simulink model "GraphicEqualizer"  (Simulink 6.6)
settings: Solver=FixedStepDiscrete  StartTime=0.0  StopTime=inf  RelTol=1e-3
PreLoadFcn:
  | Frame=64;  % number of points in a frame
InitFcn:
  | GraphicGUI
StopFcn:
  | save_system(gcs)
  | save eq_coefficients  num_den_coef
  | GraphicGUI('save_state')
undefined symbols (not defined in the file or in its folder): dfilt
libraries: dspsrcs4 x16, dsparch4 x5, simulink x2, dspwin32 x2
CloseFcn:
  | close all
settings Model: Creator=aanantha  LastModifiedBy=allways
settings DataIOCC: SaveOutput=off  SaveTime=off  SignalLoggingName=sigsOut
settings DebuggingCC: SignalResolutionControl=TryResolveAllWithWarning  SolverPrmCheckMsg=none  InheritedTsInSrcMsg=none  MultiTaskDSMMsg=warning  MultiTaskCondExecSysMsg=none  MultiTaskRateTransMsg=warning  StrictBusMsg=None
settings HardwareCC: TargetUnknown=on
settings RTWCC: IncludeERTFirstTime=on

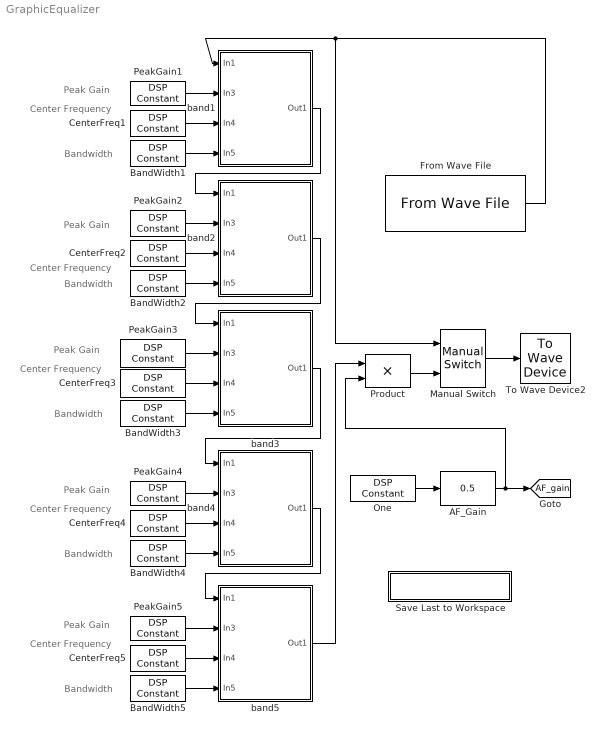
== system GraphicEqualizer ==
  note: Peak Gain
  note: Center Frequency
  note: Bandwidth
  note: Peak Gain
  note: Center Frequency
  note: Bandwidth
  note: Peak Gain
  note: Center Frequency
  note: Bandwidth
  note: Peak Gain
  note: Center Frequency
  note: Bandwidth
  note: Peak Gain
  note: Center Frequency
  note: Bandwidth
  AF_Gain : simulink/Math Operations/Slider Gain  SystemSampleTime=-1  low=0.1  gain=0.5  high=1
  BandWidth1 : dspsrcs4/DSP Constant  Tag=paramsBlock  SystemSampleTime=-1  Value=0.0071238  SampleMode=Discrete  discreteOutput=Sample-based  continuousOutput=Sample-based  sampTime=-1  framePeriod=-1  dataType=Inherit from 'Constant value'  isSigned=on  wordLen=16  udDataType=sfix(16)  fracBitsMode=Best precision  numFracBits=15  InterpretAs1D=off  Ts=-1  FramebasedOutput=off
      settings: AttributesFormatString=\n\n\n\n
  BandWidth2 : dspsrcs4/DSP Constant  Tag=paramsBlock  SystemSampleTime=-1  Value=0.070364  SampleMode=Discrete  discreteOutput=Sample-based  continuousOutput=Sample-based  sampTime=-1  framePeriod=-1  dataType=Inherit from 'Constant value'  isSigned=on  wordLen=16  udDataType=sfix(16)  fracBitsMode=Best precision  numFracBits=15  InterpretAs1D=off  Ts=-1  FramebasedOutput=off
      settings: AttributesFormatString=\n\n\n\n
  BandWidth3 : dspsrcs4/DSP Constant  Tag=paramsBlock  SystemSampleTime=-1  Value=0.66183  SampleMode=Discrete  discreteOutput=Sample-based  continuousOutput=Sample-based  sampTime=-1  framePeriod=-1  dataType=Inherit from 'Constant value'  isSigned=on  wordLen=16  udDataType=sfix(16)  fracBitsMode=Best precision  numFracBits=15  InterpretAs1D=off  Ts=-1  FramebasedOutput=off
      settings: AttributesFormatString=\n\n\n\n
  BandWidth4 : dspsrcs4/DSP Constant  Tag=paramsBlock  SystemSampleTime=-1  Value=0.44704  SampleMode=Discrete  discreteOutput=Sample-based  continuousOutput=Sample-based  sampTime=-1  framePeriod=-1  dataType=Inherit from 'Constant value'  isSigned=on  wordLen=16  udDataType=sfix(16)  fracBitsMode=Best precision  numFracBits=15  InterpretAs1D=off  Ts=-1  FramebasedOutput=off
      settings: AttributesFormatString=\n\n\n\n
  BandWidth5 : dspsrcs4/DSP Constant  Tag=paramsBlock  SystemSampleTime=-1  Value=0.039703  SampleMode=Discrete  discreteOutput=Sample-based  continuousOutput=Sample-based  sampTime=-1  framePeriod=-1  dataType=Inherit from 'Constant value'  isSigned=on  wordLen=16  udDataType=sfix(16)  fracBitsMode=Best precision  numFracBits=15  InterpretAs1D=off  Ts=-1  FramebasedOutput=off
      settings: AttributesFormatString=\n\n\n\n
  CenterFreq1 : dspsrcs4/DSP Constant  Tag=paramsBlock  SystemSampleTime=-1  Value=0.034624  SampleMode=Discrete  discreteOutput=Sample-based  continuousOutput=Sample-based  sampTime=-1  framePeriod=-1  dataType=Inherit from 'Constant value'  isSigned=on  wordLen=16  udDataType=sfix(16)  fracBitsMode=Best precision  numFracBits=15  InterpretAs1D=off  Ts=-1  FramebasedOutput=off
      settings: AttributesFormatString=\n\n\n\n
  CenterFreq2 : dspsrcs4/DSP Constant  Tag=paramsBlock  SystemSampleTime=-1  Value=0.016233  SampleMode=Discrete  discreteOutput=Sample-based  continuousOutput=Sample-based  sampTime=-1  framePeriod=-1  dataType=Inherit from 'Constant value'  isSigned=on  wordLen=16  udDataType=sfix(16)  fracBitsMode=Best precision  numFracBits=15  InterpretAs1D=off  Ts=-1  FramebasedOutput=off
      settings: AttributesFormatString=\n\n\n\n
  CenterFreq3 : dspsrcs4/DSP Constant  Tag=paramsBlock  SystemSampleTime=-1  Value=1.2233  SampleMode=Discrete  discreteOutput=Sample-based  continuousOutput=Sample-based  sampTime=-1  framePeriod=-1  dataType=Inherit from 'Constant value'  isSigned=on  wordLen=16  udDataType=sfix(16)  fracBitsMode=Best precision  numFracBits=15  InterpretAs1D=off  Ts=-1  FramebasedOutput=off
      settings: AttributesFormatString=\n\n\n\n
  CenterFreq4 : dspsrcs4/DSP Constant  Tag=paramsBlock  SystemSampleTime=-1  Value=0.88231  SampleMode=Discrete  discreteOutput=Sample-based  continuousOutput=Sample-based  sampTime=-1  framePeriod=-1  dataType=Inherit from 'Constant value'  isSigned=on  wordLen=16  udDataType=sfix(16)  fracBitsMode=Best precision  numFracBits=15  InterpretAs1D=off  Ts=-1  FramebasedOutput=off
      settings: AttributesFormatString=\n\n\n\n
  CenterFreq5 : dspsrcs4/DSP Constant  Tag=paramsBlock  SystemSampleTime=-1  Value=0.084415  SampleMode=Discrete  discreteOutput=Sample-based  continuousOutput=Sample-based  sampTime=-1  framePeriod=-1  dataType=Inherit from 'Constant value'  isSigned=on  wordLen=16  udDataType=sfix(16)  fracBitsMode=Best precision  numFracBits=15  InterpretAs1D=off  Ts=-1  FramebasedOutput=off
      settings: AttributesFormatString=\n\n\n\n
  From Wave File : dspwin32/From Wave File  FileName=HatikvahClip.wav  SamplesPerFrame=Frame  MinBufSize=256  dType=double  bLoop=on  timesToPlay=inf  restartMode=at beginning of next frame (zero pad)  firstSampleOutput=off  lastSampleOutput=off
  Manual Switch : simulink/Signal Routing/Manual Switch  SystemSampleTime=-1  sw=0  action=0  varsize=off
  One : dspsrcs4/DSP Constant  Tag=paramsBlock  SystemSampleTime=-1  Value=1  SampleMode=Discrete  discreteOutput=Sample-based  continuousOutput=Sample-based  sampTime=-1  framePeriod=-1  dataType=Inherit from 'Constant value'  isSigned=on  wordLen=16  udDataType=sfix(16)  fracBitsMode=Best precision  numFracBits=15  InterpretAs1D=off  Ts=-1  FramebasedOutput=off
      settings: AttributesFormatString=\n\n\n\n
  PeakGain1 : dspsrcs4/DSP Constant  Tag=paramsBlock  SystemSampleTime=-1  Value=-2.5998  SampleMode=Discrete  discreteOutput=Sample-based  continuousOutput=Sample-based  sampTime=-1  framePeriod=-1  dataType=Inherit from 'Constant value'  isSigned=on  wordLen=16  udDataType=sfix(16)  fracBitsMode=Best precision  numFracBits=15  InterpretAs1D=off  Ts=-1  FramebasedOutput=off
      settings: AttributesFormatString=\n\n\n\n
  PeakGain2 : dspsrcs4/DSP Constant  Tag=paramsBlock  SystemSampleTime=-1  Value=-9.6376  SampleMode=Discrete  discreteOutput=Sample-based  continuousOutput=Sample-based  sampTime=-1  framePeriod=-1  dataType=Inherit from 'Constant value'  isSigned=on  wordLen=16  udDataType=sfix(16)  fracBitsMode=Best precision  numFracBits=15  InterpretAs1D=off  Ts=-1  FramebasedOutput=off
      settings: AttributesFormatString=\n\n\n\n
  PeakGain3 : dspsrcs4/DSP Constant  Tag=paramsBlock  SystemSampleTime=-1  Value=-11.0414  SampleMode=Discrete  discreteOutput=Sample-based  continuousOutput=Sample-based  sampTime=-1  framePeriod=-1  dataType=Inherit from 'Constant value'  isSigned=on  wordLen=16  udDataType=sfix(16)  fracBitsMode=Best precision  numFracBits=15  InterpretAs1D=off  Ts=-1  FramebasedOutput=off
      settings: AttributesFormatString=\n\n\n\n
  PeakGain4 : dspsrcs4/DSP Constant  Tag=paramsBlock  SystemSampleTime=-1  Value=8.1249  SampleMode=Discrete  discreteOutput=Sample-based  continuousOutput=Sample-based  sampTime=-1  framePeriod=-1  dataType=Inherit from 'Constant value'  isSigned=on  wordLen=16  udDataType=sfix(16)  fracBitsMode=Best precision  numFracBits=15  InterpretAs1D=off  Ts=-1  FramebasedOutput=off
      settings: AttributesFormatString=\n\n\n\n
  PeakGain5 : dspsrcs4/DSP Constant  Tag=paramsBlock  SystemSampleTime=-1  Value=6.5813  SampleMode=Discrete  discreteOutput=Sample-based  continuousOutput=Sample-based  sampTime=-1  framePeriod=-1  dataType=Inherit from 'Constant value'  isSigned=on  wordLen=16  udDataType=sfix(16)  fracBitsMode=Best precision  numFracBits=15  InterpretAs1D=off  Ts=-1  FramebasedOutput=off
      settings: AttributesFormatString=\n\n\n\n
  Product : Product  SaturateOnIntegerOverflow=on
  Save Last to Workspace : Subsystem
      mask Display: disp('Save Coefficients')
  To Wave Device2 : dspwin32/To Wave Device  bufDuration=2  determineBufSize=on  userIntBufSize=256  initDelay=0.1  useDefaultDevice=off  userDeviceID=SoundMAX HD Audio  enable24Bit=off
  band1 : Subsystem  mask(Parametric Equalizer){G0=0, gbPopup=User-Defined, NdB=.707}
      mask prompts: G0 "Reference gain G0"; gbPopup "Bandwidth Gain"; NdB "Attenuation Factor (Bandwidth Gain = af*Peak Gain; 0<af<1)"
      mask help: This block contains the second order IIR filter which functions as a parametric equalizer. The Inputs to this block, in order, are the Audio In, the peak gain of the equalizer at the center frequency, the center frequency itself, and the bandwidth of the filter around the center frequency. Currently the bandedges are defined as those frequency where the gain falls off to one-half the center frequency peak gain.
      mask StyleString: edit,popup(3 dB(1/2 Power)|User-Defined),edit
      mask CallbackString: |parEqMasking|
      mask Display:
      | port_label ('input',1,'Audio In');
      | port_label ('input',2,'Peak Gain');
      | port_label ('input',3,'Center Frequency');
      | port_label ('input',4,'Bandwidth');
  band2 : Subsystem  mask(Parametric Equalizer){G0=0, gbPopup=User-Defined, NdB=.707}
      mask prompts: G0 "Reference gain G0"; gbPopup "Bandwidth Gain"; NdB "Attenuation Factor (Bandwidth Gain = af*Peak Gain; 0<af<1)"
      mask help: This block contains the second order IIR filter which functions as a parametric equalizer. The Inputs to this block, in order, are the Audio In, the peak gain of the equalizer at the center frequency, the center frequency itself, and the bandwidth of the filter around the center frequency. Currently the bandedges are defined as those frequency where the gain falls off to one-half the center frequency peak gain.
      mask StyleString: edit,popup(3 dB(1/2 Power)|User-Defined),edit
      mask CallbackString: |parEqMasking|
      mask Display:
      | port_label ('input',1,'Audio In');
      | port_label ('input',2,'Peak Gain');
      | port_label ('input',3,'Center Frequency');
      | port_label ('input',4,'Bandwidth');
  band3 : Subsystem  mask(Parametric Equalizer){G0=0, gbPopup=User-Defined, NdB=.707}
      mask prompts: G0 "Reference gain G0"; gbPopup "Bandwidth Gain"; NdB "Attenuation Factor (Bandwidth Gain = af*Peak Gain; 0<af<1)"
      mask help: This block contains the second order IIR filter which functions as a parametric equalizer. The Inputs to this block, in order, are the Audio In, the peak gain of the equalizer at the center frequency, the center frequency itself, and the bandwidth of the filter around the center frequency. Currently the bandedges are defined as those frequency where the gain falls off to one-half the center frequency peak gain.
      mask StyleString: edit,popup(3 dB(1/2 Power)|User-Defined),edit
      mask CallbackString: |parEqMasking|
      mask Display:
      | port_label ('input',1,'Audio In');
      | port_label ('input',2,'Peak Gain');
      | port_label ('input',3,'Center Frequency');
      | port_label ('input',4,'Bandwidth');
  band4 : Subsystem  mask(Parametric Equalizer){G0=0, gbPopup=User-Defined, NdB=.707}
      mask prompts: G0 "Reference gain G0"; gbPopup "Bandwidth Gain"; NdB "Attenuation Factor (Bandwidth Gain = af*Peak Gain; 0<af<1)"
      mask help: This block contains the second order IIR filter which functions as a parametric equalizer. The Inputs to this block, in order, are the Audio In, the peak gain of the equalizer at the center frequency, the center frequency itself, and the bandwidth of the filter around the center frequency. Currently the bandedges are defined as those frequency where the gain falls off to one-half the center frequency peak gain.
      mask StyleString: edit,popup(3 dB(1/2 Power)|User-Defined),edit
      mask CallbackString: |parEqMasking|
      mask Display:
      | port_label ('input',1,'Audio In');
      | port_label ('input',2,'Peak Gain');
      | port_label ('input',3,'Center Frequency');
      | port_label ('input',4,'Bandwidth');
  band5 : Subsystem  mask(Parametric Equalizer){G0=0, gbPopup=User-Defined, NdB=.707}
      mask prompts: G0 "Reference gain G0"; gbPopup "Bandwidth Gain"; NdB "Attenuation Factor (Bandwidth Gain = af*Peak Gain; 0<af<1)"
      mask help: This block contains the second order IIR filter which functions as a parametric equalizer. The Inputs to this block, in order, are the Audio In, the peak gain of the equalizer at the center frequency, the center frequency itself, and the bandwidth of the filter around the center frequency. Currently the bandedges are defined as those frequency where the gain falls off to one-half the center frequency peak gain.
      mask StyleString: edit,popup(3 dB(1/2 Power)|User-Defined),edit
      mask CallbackString: |parEqMasking|
      mask Display:
      | port_label ('input',1,'Audio In');
      | port_label ('input',2,'Peak Gain');
      | port_label ('input',3,'Center Frequency');
      | port_label ('input',4,'Bandwidth');
  tag scope: AF_gain=global
  wires:
  PeakGain2/1 -> band2/2(In3)
  CenterFreq2/1 -> band2/3(In4)
  BandWidth2/1 -> band2/4(In5)
  PeakGain3/1 -> band3/2(In3)
  CenterFreq3/1 -> band3/3(In4)
  BandWidth3/1 -> band3/4(In5)
  From Wave File/1 -> band1/1(In1), Manual Switch/1
  PeakGain1/1 -> band1/2(In3)
  CenterFreq1/1 -> band1/3(In4)
  BandWidth1/1 -> band1/4(In5)
  band1/1(Out1) -> band2/1(In1)
  band2/1(Out1) -> band3/1(In1)
  Manual Switch/1 -> To Wave Device2/1
  One/1 -> AF_Gain/1
  AF_Gain/1 -> Product/2, [AF_gain]
  Product/1 -> Manual Switch/2
  PeakGain4/1 -> band4/2(In3)
  CenterFreq4/1 -> band4/3(In4)
  BandWidth4/1 -> band4/4(In5)
  band4/1(Out1) -> band5/1(In1)
  PeakGain5/1 -> band5/2(In3)
  CenterFreq5/1 -> band5/3(In4)
  BandWidth5/1 -> band5/4(In5)
  band5/1(Out1) -> Product/1
  band3/1(Out1) -> band4/1(In1)

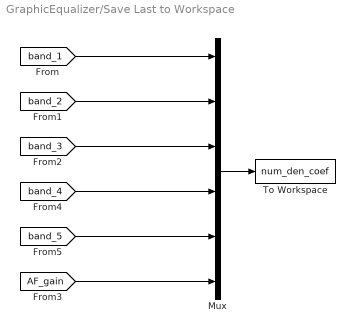
== system GraphicEqualizer/Save Last to Workspace ==
  Mux : Mux  Inputs=6
  To Workspace : ToWorkspace  VariableName=num_den_coef  SampleTime=-1  SaveFormat=Array
      settings: MaxDataPoints=1
  wires:
  [band_2] -> Mux/2
  [band_1] -> Mux/1
  [band_3] -> Mux/3
  Mux/1 -> To Workspace/1
  [band_4] -> Mux/4
  [AF_gain] -> Mux/6
  [band_5] -> Mux/5

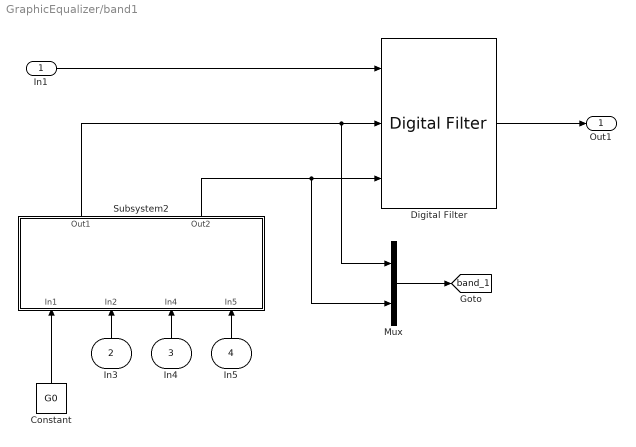
== system GraphicEqualizer/band1 ==
  In1 : Inport
  In3 : Inport  Orientation=up  Port=2
  In4 : Inport  Orientation=up  Port=3
  In5 : Inport  Orientation=up  Port=4
  Constant : Constant  Orientation=up  Value=G0
  Digital Filter : dsparch4/Digital Filter  DialogController=dspdialog.DigitalFilter  DialogControllerArgs=DataTag0  TypePopup=IIR (poles & zeros)  IIRFiltStruct=Direct form II transposed  AllPoleFiltStruct=Direct form  FIRFiltStruct=Direct form  CoeffSource=Input port(s)  NumCoeffs=[1 2]  DenCoeffs=[1 0.1]  BiQuadCoeffs=[1 0.3 0.4 1 0.1 0.2]  LatticeCoeffs=[0.2 0.4]  denIgnore=on  FiltPerSampPopup=One filter per frame  IC=0  ICnum=0  ICden=0  roundingMode=Floor  overflowMode=off  ScaleValues=1  scaleValueFracLength=14  stageInFracLength=15  stageOutFracLength=15  FilterSource=Input port(s)  dfiltObjectName=dfilt.dffir([1 2 1])
  Mux : Mux  Inputs=2
  Subsystem2 : Subsystem  Orientation=up
      mask Display:
      | disp('ParEq')
      | port_label('input',1,'G0');
      | port_label('input',2,'G');
      | port_label('input',3,'w0');
      | port_label('input',4,'Dw');
      | 
      | port_label('output',1,'Num');
      | port_label('output',2,'Den');
  Out1 : Outport
  tag scope: band_1=global
  wires:
  Subsystem2/1(Out1) -> Digital Filter/2, Mux/1
  Subsystem2/2(Out2) -> Digital Filter/3, Mux/2
  In1/1 -> Digital Filter/1
  Digital Filter/1 -> Out1/1
  In3/1 -> Subsystem2/2(In2)
  In4/1 -> Subsystem2/3(In4)
  In5/1 -> Subsystem2/4(In5)
  Constant/1 -> Subsystem2/1(In1)
  Mux/1 -> [band_1]

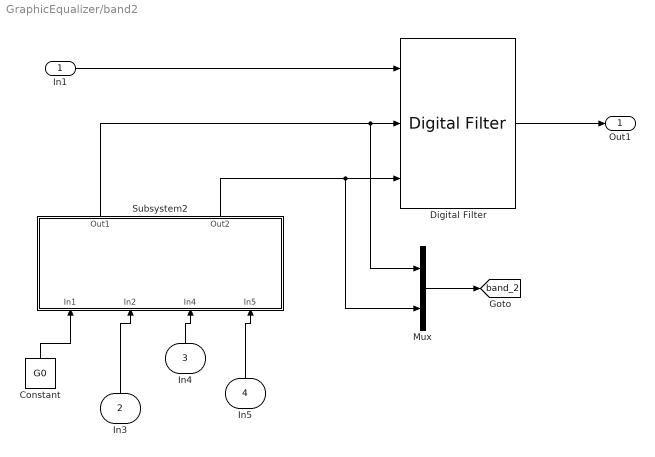
== system GraphicEqualizer/band2 ==
  In1 : Inport
  In3 : Inport  Orientation=up  Port=2
  In4 : Inport  Orientation=up  Port=3
  In5 : Inport  Orientation=up  Port=4
  Constant : Constant  Orientation=up  Value=G0
  Digital Filter : dsparch4/Digital Filter  DialogController=dspdialog.DigitalFilter  DialogControllerArgs=DataTag1  TypePopup=IIR (poles & zeros)  IIRFiltStruct=Direct form II transposed  AllPoleFiltStruct=Direct form  FIRFiltStruct=Direct form  CoeffSource=Input port(s)  NumCoeffs=[1 2]  DenCoeffs=[1 0.1]  BiQuadCoeffs=[1 0.3 0.4 1 0.1 0.2]  LatticeCoeffs=[0.2 0.4]  denIgnore=on  FiltPerSampPopup=One filter per frame  IC=0  ICnum=0  ICden=0  roundingMode=Floor  overflowMode=off  ScaleValues=1  scaleValueFracLength=14  stageInFracLength=15  stageOutFracLength=15  FilterSource=Input port(s)  dfiltObjectName=dfilt.dffir([1 2 1])
  Mux : Mux  Inputs=2
  Subsystem2 : Subsystem  Orientation=up
      mask Display:
      | disp('ParEq')
      | port_label('input',1,'G0');
      | port_label('input',2,'G');
      | port_label('input',3,'w0');
      | port_label('input',4,'Dw');
      | 
      | port_label('output',1,'Num');
      | port_label('output',2,'Den');
  Out1 : Outport
  tag scope: band_2=global
  wires:
  Constant/1 -> Subsystem2/1(In1)
  In5/1 -> Subsystem2/4(In5)
  In4/1 -> Subsystem2/3(In4)
  In3/1 -> Subsystem2/2(In2)
  Digital Filter/1 -> Out1/1
  In1/1 -> Digital Filter/1
  Subsystem2/2(Out2) -> Digital Filter/3, Mux/2
  Subsystem2/1(Out1) -> Digital Filter/2, Mux/1
  Mux/1 -> [band_2]

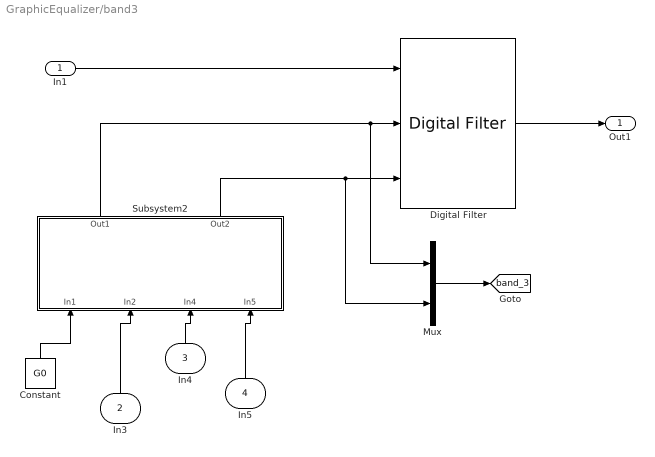
== system GraphicEqualizer/band3 ==
  In1 : Inport
  In3 : Inport  Orientation=up  Port=2
  In4 : Inport  Orientation=up  Port=3
  In5 : Inport  Orientation=up  Port=4
  Constant : Constant  Orientation=up  Value=G0
  Digital Filter : dsparch4/Digital Filter  DialogController=dspdialog.DigitalFilter  DialogControllerArgs=DataTag2  TypePopup=IIR (poles & zeros)  IIRFiltStruct=Direct form II transposed  AllPoleFiltStruct=Direct form  FIRFiltStruct=Direct form  CoeffSource=Input port(s)  NumCoeffs=[1 2]  DenCoeffs=[1 0.1]  BiQuadCoeffs=[1 0.3 0.4 1 0.1 0.2]  LatticeCoeffs=[0.2 0.4]  denIgnore=on  FiltPerSampPopup=One filter per frame  IC=0  ICnum=0  ICden=0  roundingMode=Floor  overflowMode=off  ScaleValues=1  scaleValueFracLength=14  stageInFracLength=15  stageOutFracLength=15  FilterSource=Input port(s)  dfiltObjectName=dfilt.dffir([1 2 1])
  Mux : Mux  Inputs=2
  Subsystem2 : Subsystem  Orientation=up
      mask Display:
      | disp('ParEq')
      | port_label('input',1,'G0');
      | port_label('input',2,'G');
      | port_label('input',3,'w0');
      | port_label('input',4,'Dw');
      | 
      | port_label('output',1,'Num');
      | port_label('output',2,'Den');
  Out1 : Outport
  tag scope: band_3=global
  wires:
  Subsystem2/1(Out1) -> Digital Filter/2, Mux/1
  Subsystem2/2(Out2) -> Digital Filter/3, Mux/2
  In1/1 -> Digital Filter/1
  Digital Filter/1 -> Out1/1
  In3/1 -> Subsystem2/2(In2)
  In4/1 -> Subsystem2/3(In4)
  In5/1 -> Subsystem2/4(In5)
  Constant/1 -> Subsystem2/1(In1)
  Mux/1 -> [band_3]

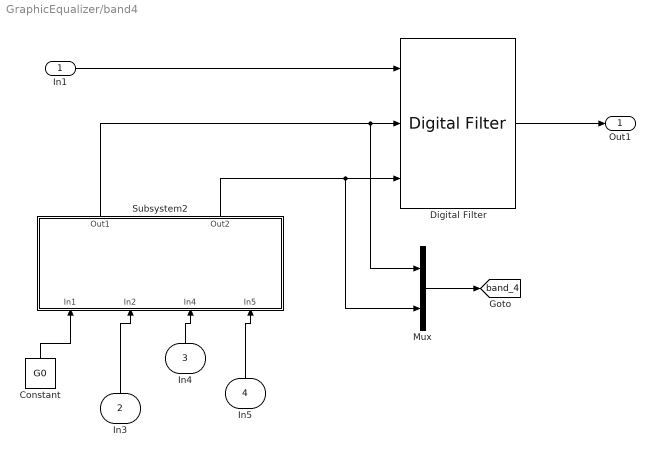
== system GraphicEqualizer/band4 ==
  In1 : Inport
  In3 : Inport  Orientation=up  Port=2
  In4 : Inport  Orientation=up  Port=3
  In5 : Inport  Orientation=up  Port=4
  Constant : Constant  Orientation=up  Value=G0
  Digital Filter : dsparch4/Digital Filter  DialogController=dspdialog.DigitalFilter  DialogControllerArgs=DataTag3  TypePopup=IIR (poles & zeros)  IIRFiltStruct=Direct form II transposed  AllPoleFiltStruct=Direct form  FIRFiltStruct=Direct form  CoeffSource=Input port(s)  NumCoeffs=[1 2]  DenCoeffs=[1 0.1]  BiQuadCoeffs=[1 0.3 0.4 1 0.1 0.2]  LatticeCoeffs=[0.2 0.4]  denIgnore=on  FiltPerSampPopup=One filter per frame  IC=0  ICnum=0  ICden=0  roundingMode=Floor  overflowMode=off  ScaleValues=1  scaleValueFracLength=14  stageInFracLength=15  stageOutFracLength=15  FilterSource=Input port(s)  dfiltObjectName=dfilt.dffir([1 2 1])
  Mux : Mux  Inputs=2
  Subsystem2 : Subsystem  Orientation=up
      mask Display:
      | disp('ParEq')
      | port_label('input',1,'G0');
      | port_label('input',2,'G');
      | port_label('input',3,'w0');
      | port_label('input',4,'Dw');
      | 
      | port_label('output',1,'Num');
      | port_label('output',2,'Den');
  Out1 : Outport
  tag scope: band_4=global
  wires:
  Constant/1 -> Subsystem2/1(In1)
  In5/1 -> Subsystem2/4(In5)
  In4/1 -> Subsystem2/3(In4)
  In3/1 -> Subsystem2/2(In2)
  Digital Filter/1 -> Out1/1
  In1/1 -> Digital Filter/1
  Subsystem2/2(Out2) -> Digital Filter/3, Mux/2
  Subsystem2/1(Out1) -> Digital Filter/2, Mux/1
  Mux/1 -> [band_4]

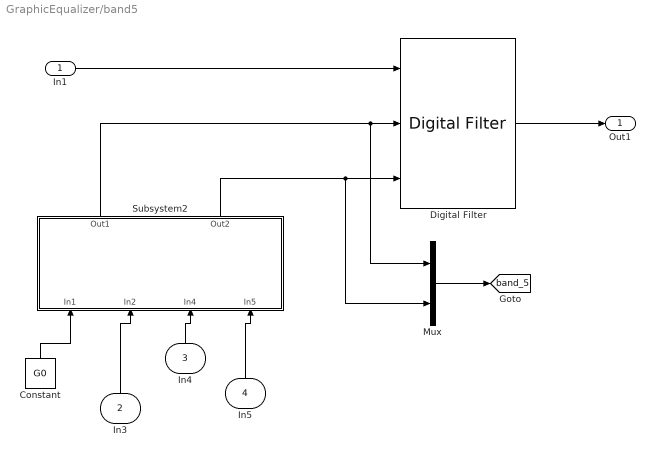
== system GraphicEqualizer/band5 ==
  In1 : Inport
  In3 : Inport  Orientation=up  Port=2
  In4 : Inport  Orientation=up  Port=3
  In5 : Inport  Orientation=up  Port=4
  Constant : Constant  Orientation=up  Value=G0
  Digital Filter : dsparch4/Digital Filter  DialogController=dspdialog.DigitalFilter  DialogControllerArgs=DataTag4  TypePopup=IIR (poles & zeros)  IIRFiltStruct=Direct form II transposed  AllPoleFiltStruct=Direct form  FIRFiltStruct=Direct form  CoeffSource=Input port(s)  NumCoeffs=[1 2]  DenCoeffs=[1 0.1]  BiQuadCoeffs=[1 0.3 0.4 1 0.1 0.2]  LatticeCoeffs=[0.2 0.4]  denIgnore=on  FiltPerSampPopup=One filter per frame  IC=0  ICnum=0  ICden=0  roundingMode=Floor  overflowMode=off  ScaleValues=1  scaleValueFracLength=14  stageInFracLength=15  stageOutFracLength=15  FilterSource=Input port(s)  dfiltObjectName=dfilt.dffir([1 2 1])
  Mux : Mux  Inputs=2
  Subsystem2 : Subsystem  Orientation=up
      mask Display:
      | disp('ParEq')
      | port_label('input',1,'G0');
      | port_label('input',2,'G');
      | port_label('input',3,'w0');
      | port_label('input',4,'Dw');
      | 
      | port_label('output',1,'Num');
      | port_label('output',2,'Den');
  Out1 : Outport
  tag scope: band_5=global
  wires:
  Subsystem2/1(Out1) -> Digital Filter/2, Mux/1
  Subsystem2/2(Out2) -> Digital Filter/3, Mux/2
  In1/1 -> Digital Filter/1
  Digital Filter/1 -> Out1/1
  In3/1 -> Subsystem2/2(In2)
  In4/1 -> Subsystem2/3(In4)
  In5/1 -> Subsystem2/4(In5)
  Constant/1 -> Subsystem2/1(In1)
  Mux/1 -> [band_5]

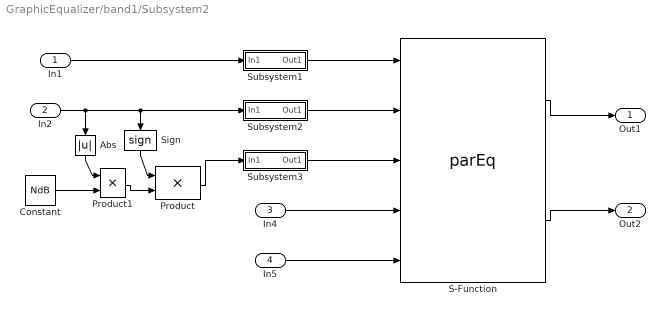
== system GraphicEqualizer/band1/Subsystem2 ==
  In1 : Inport
  In2 : Inport  Port=2
  In4 : Inport  Port=3
  In5 : Inport  Port=4
  Abs : Abs  Orientation=down  SaturateOnIntegerOverflow=on
  Constant : Constant  Value=NdB
  Product : Product  SaturateOnIntegerOverflow=on
  Product1 : Product  SaturateOnIntegerOverflow=on
  S-Function : S-Function  FunctionName=parEq
      mask Type: Parametric Equalizer Coefficients
      mask Description: Generate the filter coefficients based on the band values.
      mask Help: Based on Parametric Equalizer filter design by Orfanidis.
      mask Display:
      | disp('ParEq')
      | port_label('input',1,'G0');
      | port_label('input',2,'G');
      | port_label('input',3,'GB');
      | port_label('input',4,'w0');
      | port_label('input',5,'Dw');
      | 
      | port_label('output',1,'Num');
      | port_label('output',2,'Den');
  Sign : Signum  Orientation=down
  Subsystem1 : Subsystem
      mask Type: DbtoReal
      mask Description: Converts inputs in dB to real values. Formula --> 10^(u/20)
      mask Display: disp('dB->Real')
  Subsystem2 : Subsystem
      mask Type: DbtoReal
      mask Description: Converts inputs in dB to real values. Formula --> 10^(u/20)
      mask Display: disp('dB->Real')
  Subsystem3 : Subsystem
      mask Type: DbtoReal
      mask Description: Converts inputs in dB to real values. Formula --> 10^(u/20)
      mask Display: disp('dB->Real')
  Out1 : Outport
  Out2 : Outport  Port=2
  wires:
  In5/1 -> S-Function/5
  S-Function/2 -> Out2/1
  In4/1 -> S-Function/4
  In2/1 -> Abs/1, Subsystem2/1(In1), Sign/1
  S-Function/1 -> Out1/1
  In1/1 -> Subsystem1/1(In1)
  Subsystem3/1(Out1) -> S-Function/3
  Subsystem2/1(Out1) -> S-Function/2
  Subsystem1/1(Out1) -> S-Function/1
  Constant/1 -> Product1/2
  Abs/1 -> Product1/1
  Product1/1 -> Product/2
  Sign/1 -> Product/1
  Product/1 -> Subsystem3/1(In1)

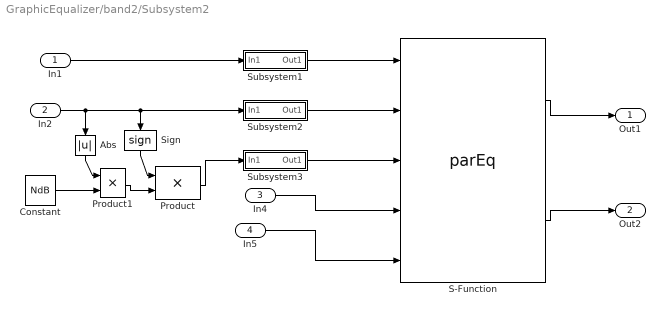
== system GraphicEqualizer/band2/Subsystem2 ==
  In1 : Inport
  In2 : Inport  Port=2
  In4 : Inport  Port=3
  In5 : Inport  Port=4
  Abs : Abs  Orientation=down  SaturateOnIntegerOverflow=on
  Constant : Constant  Value=NdB
  Product : Product  SaturateOnIntegerOverflow=on
  Product1 : Product  SaturateOnIntegerOverflow=on
  S-Function : S-Function  FunctionName=parEq
      mask Type: Parametric Equalizer Coefficients
      mask Description: Generate the filter coefficients based on the band values.
      mask Help: Based on Parametric Equalizer filter design by Orfanidis.
      mask Display:
      | disp('ParEq')
      | port_label('input',1,'G0');
      | port_label('input',2,'G');
      | port_label('input',3,'GB');
      | port_label('input',4,'w0');
      | port_label('input',5,'Dw');
      | 
      | port_label('output',1,'Num');
      | port_label('output',2,'Den');
  Sign : Signum  Orientation=down
  Subsystem1 : Subsystem
      mask Type: DbtoReal
      mask Description: Converts inputs in dB to real values. Formula --> 10^(u/20)
      mask Display: disp('dB->Real')
  Subsystem2 : Subsystem
      mask Type: DbtoReal
      mask Description: Converts inputs in dB to real values. Formula --> 10^(u/20)
      mask Display: disp('dB->Real')
  Subsystem3 : Subsystem
      mask Type: DbtoReal
      mask Description: Converts inputs in dB to real values. Formula --> 10^(u/20)
      mask Display: disp('dB->Real')
  Out1 : Outport
  Out2 : Outport  Port=2
  wires:
  Product/1 -> Subsystem3/1(In1)
  Sign/1 -> Product/1
  Product1/1 -> Product/2
  Abs/1 -> Product1/1
  Constant/1 -> Product1/2
  Subsystem1/1(Out1) -> S-Function/1
  Subsystem2/1(Out1) -> S-Function/2
  Subsystem3/1(Out1) -> S-Function/3
  In1/1 -> Subsystem1/1(In1)
  S-Function/1 -> Out1/1
  In2/1 -> Sign/1, Subsystem2/1(In1), Abs/1
  In4/1 -> S-Function/4
  S-Function/2 -> Out2/1
  In5/1 -> S-Function/5

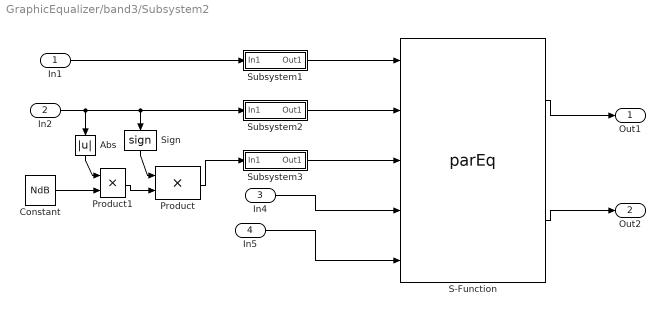
== system GraphicEqualizer/band3/Subsystem2 ==
  In1 : Inport
  In2 : Inport  Port=2
  In4 : Inport  Port=3
  In5 : Inport  Port=4
  Abs : Abs  Orientation=down  SaturateOnIntegerOverflow=on
  Constant : Constant  Value=NdB
  Product : Product  SaturateOnIntegerOverflow=on
  Product1 : Product  SaturateOnIntegerOverflow=on
  S-Function : S-Function  FunctionName=parEq
      mask Type: Parametric Equalizer Coefficients
      mask Description: Generate the filter coefficients based on the band values.
      mask Help: Based on Parametric Equalizer filter design by Orfanidis.
      mask Display:
      | disp('ParEq')
      | port_label('input',1,'G0');
      | port_label('input',2,'G');
      | port_label('input',3,'GB');
      | port_label('input',4,'w0');
      | port_label('input',5,'Dw');
      | 
      | port_label('output',1,'Num');
      | port_label('output',2,'Den');
  Sign : Signum  Orientation=down
  Subsystem1 : Subsystem
      mask Type: DbtoReal
      mask Description: Converts inputs in dB to real values. Formula --> 10^(u/20)
      mask Display: disp('dB->Real')
  Subsystem2 : Subsystem
      mask Type: DbtoReal
      mask Description: Converts inputs in dB to real values. Formula --> 10^(u/20)
      mask Display: disp('dB->Real')
  Subsystem3 : Subsystem
      mask Type: DbtoReal
      mask Description: Converts inputs in dB to real values. Formula --> 10^(u/20)
      mask Display: disp('dB->Real')
  Out1 : Outport
  Out2 : Outport  Port=2
  wires:
  In5/1 -> S-Function/5
  S-Function/2 -> Out2/1
  In4/1 -> S-Function/4
  In2/1 -> Abs/1, Subsystem2/1(In1), Sign/1
  S-Function/1 -> Out1/1
  In1/1 -> Subsystem1/1(In1)
  Subsystem3/1(Out1) -> S-Function/3
  Subsystem2/1(Out1) -> S-Function/2
  Subsystem1/1(Out1) -> S-Function/1
  Constant/1 -> Product1/2
  Abs/1 -> Product1/1
  Product1/1 -> Product/2
  Sign/1 -> Product/1
  Product/1 -> Subsystem3/1(In1)

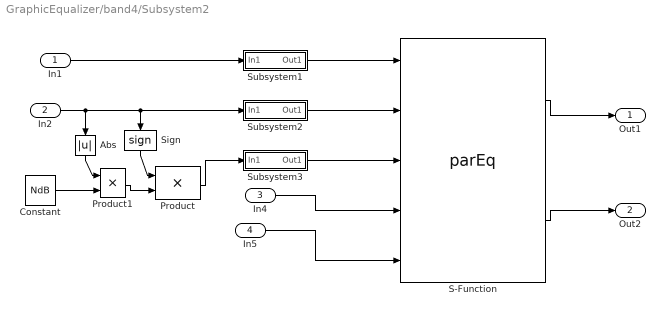
== system GraphicEqualizer/band4/Subsystem2 ==
  In1 : Inport
  In2 : Inport  Port=2
  In4 : Inport  Port=3
  In5 : Inport  Port=4
  Abs : Abs  Orientation=down  SaturateOnIntegerOverflow=on
  Constant : Constant  Value=NdB
  Product : Product  SaturateOnIntegerOverflow=on
  Product1 : Product  SaturateOnIntegerOverflow=on
  S-Function : S-Function  FunctionName=parEq
      mask Type: Parametric Equalizer Coefficients
      mask Description: Generate the filter coefficients based on the band values.
      mask Help: Based on Parametric Equalizer filter design by Orfanidis.
      mask Display:
      | disp('ParEq')
      | port_label('input',1,'G0');
      | port_label('input',2,'G');
      | port_label('input',3,'GB');
      | port_label('input',4,'w0');
      | port_label('input',5,'Dw');
      | 
      | port_label('output',1,'Num');
      | port_label('output',2,'Den');
  Sign : Signum  Orientation=down
  Subsystem1 : Subsystem
      mask Type: DbtoReal
      mask Description: Converts inputs in dB to real values. Formula --> 10^(u/20)
      mask Display: disp('dB->Real')
  Subsystem2 : Subsystem
      mask Type: DbtoReal
      mask Description: Converts inputs in dB to real values. Formula --> 10^(u/20)
      mask Display: disp('dB->Real')
  Subsystem3 : Subsystem
      mask Type: DbtoReal
      mask Description: Converts inputs in dB to real values. Formula --> 10^(u/20)
      mask Display: disp('dB->Real')
  Out1 : Outport
  Out2 : Outport  Port=2
  wires:
  Product/1 -> Subsystem3/1(In1)
  Sign/1 -> Product/1
  Product1/1 -> Product/2
  Abs/1 -> Product1/1
  Constant/1 -> Product1/2
  Subsystem1/1(Out1) -> S-Function/1
  Subsystem2/1(Out1) -> S-Function/2
  Subsystem3/1(Out1) -> S-Function/3
  In1/1 -> Subsystem1/1(In1)
  S-Function/1 -> Out1/1
  In2/1 -> Sign/1, Subsystem2/1(In1), Abs/1
  In4/1 -> S-Function/4
  S-Function/2 -> Out2/1
  In5/1 -> S-Function/5

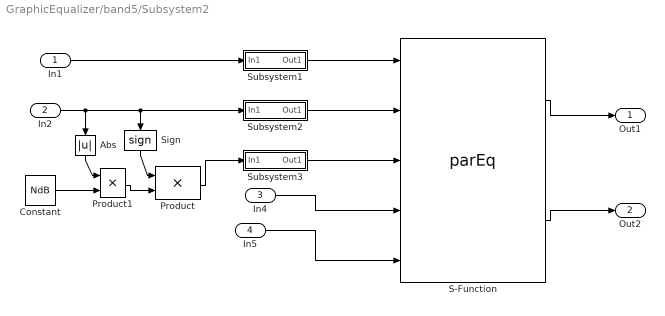
== system GraphicEqualizer/band5/Subsystem2 ==
  In1 : Inport
  In2 : Inport  Port=2
  In4 : Inport  Port=3
  In5 : Inport  Port=4
  Abs : Abs  Orientation=down  SaturateOnIntegerOverflow=on
  Constant : Constant  Value=NdB
  Product : Product  SaturateOnIntegerOverflow=on
  Product1 : Product  SaturateOnIntegerOverflow=on
  S-Function : S-Function  FunctionName=parEq
      mask Type: Parametric Equalizer Coefficients
      mask Description: Generate the filter coefficients based on the band values.
      mask Help: Based on Parametric Equalizer filter design by Orfanidis.
      mask Display:
      | disp('ParEq')
      | port_label('input',1,'G0');
      | port_label('input',2,'G');
      | port_label('input',3,'GB');
      | port_label('input',4,'w0');
      | port_label('input',5,'Dw');
      | 
      | port_label('output',1,'Num');
      | port_label('output',2,'Den');
  Sign : Signum  Orientation=down
  Subsystem1 : Subsystem
      mask Type: DbtoReal
      mask Description: Converts inputs in dB to real values. Formula --> 10^(u/20)
      mask Display: disp('dB->Real')
  Subsystem2 : Subsystem
      mask Type: DbtoReal
      mask Description: Converts inputs in dB to real values. Formula --> 10^(u/20)
      mask Display: disp('dB->Real')
  Subsystem3 : Subsystem
      mask Type: DbtoReal
      mask Description: Converts inputs in dB to real values. Formula --> 10^(u/20)
      mask Display: disp('dB->Real')
  Out1 : Outport
  Out2 : Outport  Port=2
  wires:
  In5/1 -> S-Function/5
  S-Function/2 -> Out2/1
  In4/1 -> S-Function/4
  In2/1 -> Abs/1, Subsystem2/1(In1), Sign/1
  S-Function/1 -> Out1/1
  In1/1 -> Subsystem1/1(In1)
  Subsystem3/1(Out1) -> S-Function/3
  Subsystem2/1(Out1) -> S-Function/2
  Subsystem1/1(Out1) -> S-Function/1
  Constant/1 -> Product1/2
  Abs/1 -> Product1/1
  Product1/1 -> Product/2
  Sign/1 -> Product/1
  Product/1 -> Subsystem3/1(In1)

== system GraphicEqualizer/band1/Subsystem2/Subsystem1 ==
  In1 : Inport
  Gain1 : Gain  Gain=1/20  SaturateOnIntegerOverflow=on
  Math Function : Math  Operator=10^u  OutputSignalType=real  SaturateOnIntegerOverflow=on
  Out1 : Outport
  wires:
  Gain1/1 -> Math Function/1
  In1/1 -> Gain1/1
  Math Function/1 -> Out1/1

== system GraphicEqualizer/band1/Subsystem2/Subsystem2 ==
  In1 : Inport
  Gain1 : Gain  Gain=1/20  SaturateOnIntegerOverflow=on
  Math Function : Math  Operator=10^u  OutputSignalType=real  SaturateOnIntegerOverflow=on
  Out1 : Outport
  wires:
  Math Function/1 -> Out1/1
  In1/1 -> Gain1/1
  Gain1/1 -> Math Function/1

== system GraphicEqualizer/band1/Subsystem2/Subsystem3 ==
  In1 : Inport
  Gain1 : Gain  Gain=1/20  SaturateOnIntegerOverflow=on
  Math Function : Math  Operator=10^u  OutputSignalType=real  SaturateOnIntegerOverflow=on
  Out1 : Outport
  wires:
  Gain1/1 -> Math Function/1
  In1/1 -> Gain1/1
  Math Function/1 -> Out1/1

== system GraphicEqualizer/band2/Subsystem2/Subsystem1 ==
  In1 : Inport
  Gain1 : Gain  Gain=1/20  SaturateOnIntegerOverflow=on
  Math Function : Math  Operator=10^u  OutputSignalType=real  SaturateOnIntegerOverflow=on
  Out1 : Outport
  wires:
  Math Function/1 -> Out1/1
  In1/1 -> Gain1/1
  Gain1/1 -> Math Function/1

== system GraphicEqualizer/band2/Subsystem2/Subsystem2 ==
  In1 : Inport
  Gain1 : Gain  Gain=1/20  SaturateOnIntegerOverflow=on
  Math Function : Math  Operator=10^u  OutputSignalType=real  SaturateOnIntegerOverflow=on
  Out1 : Outport
  wires:
  Gain1/1 -> Math Function/1
  In1/1 -> Gain1/1
  Math Function/1 -> Out1/1

== system GraphicEqualizer/band2/Subsystem2/Subsystem3 ==
  In1 : Inport
  Gain1 : Gain  Gain=1/20  SaturateOnIntegerOverflow=on
  Math Function : Math  Operator=10^u  OutputSignalType=real  SaturateOnIntegerOverflow=on
  Out1 : Outport
  wires:
  Math Function/1 -> Out1/1
  In1/1 -> Gain1/1
  Gain1/1 -> Math Function/1

== system GraphicEqualizer/band3/Subsystem2/Subsystem1 ==
  In1 : Inport
  Gain1 : Gain  Gain=1/20  SaturateOnIntegerOverflow=on
  Math Function : Math  Operator=10^u  OutputSignalType=real  SaturateOnIntegerOverflow=on
  Out1 : Outport
  wires:
  Gain1/1 -> Math Function/1
  In1/1 -> Gain1/1
  Math Function/1 -> Out1/1

== system GraphicEqualizer/band3/Subsystem2/Subsystem2 ==
  In1 : Inport
  Gain1 : Gain  Gain=1/20  SaturateOnIntegerOverflow=on
  Math Function : Math  Operator=10^u  OutputSignalType=real  SaturateOnIntegerOverflow=on
  Out1 : Outport
  wires:
  Math Function/1 -> Out1/1
  In1/1 -> Gain1/1
  Gain1/1 -> Math Function/1

== system GraphicEqualizer/band3/Subsystem2/Subsystem3 ==
  In1 : Inport
  Gain1 : Gain  Gain=1/20  SaturateOnIntegerOverflow=on
  Math Function : Math  Operator=10^u  OutputSignalType=real  SaturateOnIntegerOverflow=on
  Out1 : Outport
  wires:
  Gain1/1 -> Math Function/1
  In1/1 -> Gain1/1
  Math Function/1 -> Out1/1

== system GraphicEqualizer/band4/Subsystem2/Subsystem1 ==
  In1 : Inport
  Gain1 : Gain  Gain=1/20  SaturateOnIntegerOverflow=on
  Math Function : Math  Operator=10^u  OutputSignalType=real  SaturateOnIntegerOverflow=on
  Out1 : Outport
  wires:
  Math Function/1 -> Out1/1
  In1/1 -> Gain1/1
  Gain1/1 -> Math Function/1

== system GraphicEqualizer/band4/Subsystem2/Subsystem2 ==
  In1 : Inport
  Gain1 : Gain  Gain=1/20  SaturateOnIntegerOverflow=on
  Math Function : Math  Operator=10^u  OutputSignalType=real  SaturateOnIntegerOverflow=on
  Out1 : Outport
  wires:
  Gain1/1 -> Math Function/1
  In1/1 -> Gain1/1
  Math Function/1 -> Out1/1

== system GraphicEqualizer/band4/Subsystem2/Subsystem3 ==
  In1 : Inport
  Gain1 : Gain  Gain=1/20  SaturateOnIntegerOverflow=on
  Math Function : Math  Operator=10^u  OutputSignalType=real  SaturateOnIntegerOverflow=on
  Out1 : Outport
  wires:
  Math Function/1 -> Out1/1
  In1/1 -> Gain1/1
  Gain1/1 -> Math Function/1

== system GraphicEqualizer/band5/Subsystem2/Subsystem1 ==
  In1 : Inport
  Gain1 : Gain  Gain=1/20  SaturateOnIntegerOverflow=on
  Math Function : Math  Operator=10^u  OutputSignalType=real  SaturateOnIntegerOverflow=on
  Out1 : Outport
  wires:
  Gain1/1 -> Math Function/1
  In1/1 -> Gain1/1
  Math Function/1 -> Out1/1

== system GraphicEqualizer/band5/Subsystem2/Subsystem2 ==
  In1 : Inport
  Gain1 : Gain  Gain=1/20  SaturateOnIntegerOverflow=on
  Math Function : Math  Operator=10^u  OutputSignalType=real  SaturateOnIntegerOverflow=on
  Out1 : Outport
  wires:
  Math Function/1 -> Out1/1
  In1/1 -> Gain1/1
  Gain1/1 -> Math Function/1

== system GraphicEqualizer/band5/Subsystem2/Subsystem3 ==
  In1 : Inport
  Gain1 : Gain  Gain=1/20  SaturateOnIntegerOverflow=on
  Math Function : Math  Operator=10^u  OutputSignalType=real  SaturateOnIntegerOverflow=on
  Out1 : Outport
  wires:
  Gain1/1 -> Math Function/1
  In1/1 -> Gain1/1
  Math Function/1 -> Out1/1
